simulink model "lab3"  (Simulink 7.6)
settings: Solver=ode45  StartTime=0.0  StopTime=30.0  RelTol=1e-3
undefined symbols (not defined in the file): A, B, C, D
settings Model: Creator=m135982  LastModifiedBy=m135982
settings DataIOCC: LimitDataPoints=off  Refine=1000

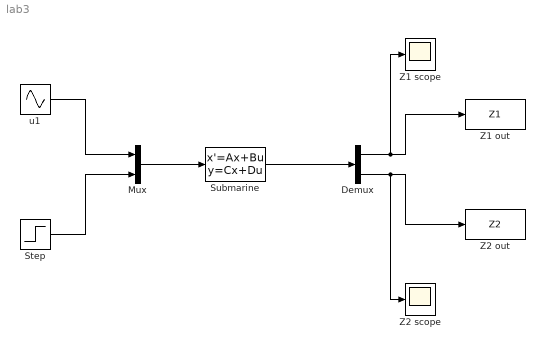
== system lab3 ==
  Demux : Demux  Outputs=2
  Mux : Mux  Inputs=2
  Step : Step  After=.1  SampleTime=0
  Submarine : StateSpace  A=A  B=B  C=C  D=D  X0=[-.1,0,.1,0]
  Z1 out : ToWorkspace  VariableName=Z1  SampleTime=-1  SaveFormat=Array
  Z1 scope : Scope
  Z2 out : ToWorkspace  VariableName=Z2  SampleTime=-1  SaveFormat=Array
  Z2 scope : Scope
  u1 : Sin  Frequency=7  SampleTime=0
  wires:
  u1/1 -> Mux/1
  Step/1 -> Mux/2
  Mux/1 -> Submarine/1
  Submarine/1 -> Demux/1
  Demux/1 -> Z1 out/1, Z1 scope/1
  Demux/2 -> Z2 out/1, Z2 scope/1
